simulink model "double_integrator"  (R2025b)
settings: Solver=FixedStepAuto  StartTime=0.0  StopTime=10.0  FixedStep=0.02  RelTol=1e-3
settings Model: Creator=Junch  LastModifiedBy=Junch

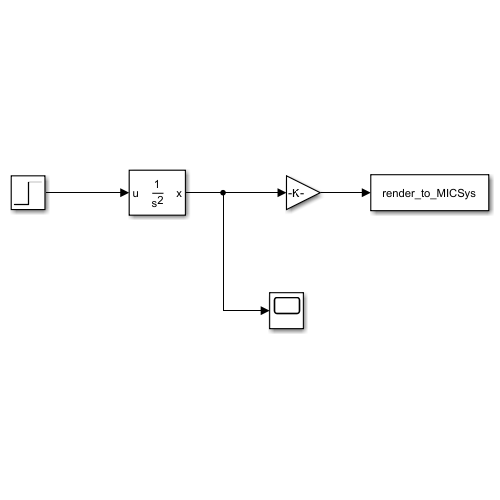
[thumbnail: Simulink's stored preview of the top-level diagram]
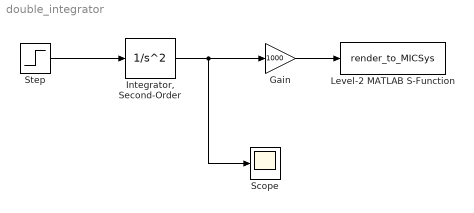
== system double_integrator ==
  Gain : Gain  Gain=1000
  "Integrator, Second-Order" : SecondOrderIntegrator  ShowOutput=x
  Level-2 MATLAB S-Function : M-S-Function  FunctionName=render_to_MICSys
  Scope : Scope
      settings: ActiveDisplayYMinimum=-14.584263144301193  ActiveDisplayYMaximum=47.434279423180136
  Step : Step  SampleTime=0
  wires:
  Step/1 -> "Integrator, Second-Order"/1
  "Integrator, Second-Order"/1 -> Scope/1, Gain/1
  Gain/1 -> Level-2 MATLAB S-Function/1
